simulink model "chua_sim"  (R2022b)
settings: Solver=ode23t  StartTime=0.0  StopTime=Tfin  RelTol=1e-3
values from neighbouring files (symbols this model uses):
  x0 = randn(3,1)*0.2    [main_chua.m]
  xp0 = x0+[0.01;0;0]    [main_chua.m]
undefined symbols (not defined in the file or in its folder): fg_chua
settings Model: Creator=carlonovara  LastModifiedBy=Enf
settings SolverCC: AlgebraicLoopSolver=TrustRegion
settings DataIOCC: ReturnWorkspaceOutputs=off
settings DebuggingCC: UnconnectedInputMsg=warning  UnconnectedOutputMsg=warning  UnconnectedLineMsg=warning  SFMachineParentedDataDiag=warning  ArithmeticOperatorsInVariantConditions=warning
settings ModelReferenceCC: EnableRefExpFcnMdlSchedulingChecks=on
settings SFSimCC: SimUseLocalCustomCode=off  CustomCodeUndefinedFunction=UseInterfaceOnly
settings RTWCC: RTWUseLocalCustomCode=off
settings CodeAppCC: StateflowObjectComments=on

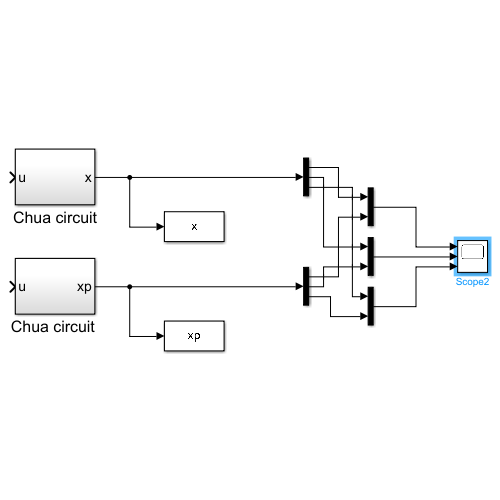
[thumbnail: Simulink's stored preview of the top-level diagram]
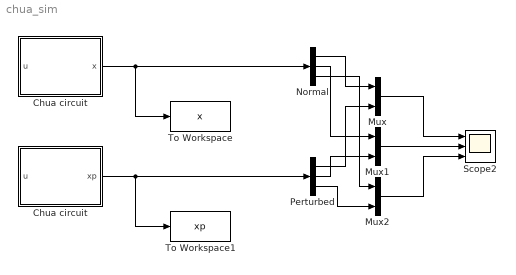
== system chua_sim ==
  Chua circuit : Subsystem
  "Chua circuit " : Subsystem
  Mux : Mux  Inputs=2
  Mux1 : Mux  Inputs=2
  Mux2 : Mux  Inputs=2
  Normal : Demux  Outputs=3
  Perturbed : Demux  Outputs=3
  Scope2 : Scope  NumInputPorts=3
  To Workspace : ToWorkspace  VariableName=x  SampleTime=-1
  To Workspace1 : ToWorkspace  VariableName=xp  SampleTime=-1
  wires:
  Chua circuit/1(x) -> To Workspace/1, Normal/1
  "Chua circuit "/1(xp) -> To Workspace1/1, Perturbed/1
  Mux/1 -> Scope2/1
  Mux1/1 -> Scope2/2
  Mux2/1 -> Scope2/3
  Normal/1 -> Mux/1
  Perturbed/1 -> Mux/2
  Normal/2 -> Mux1/1
  Perturbed/2 -> Mux1/2
  Normal/3 -> Mux2/1
  Perturbed/3 -> Mux2/2

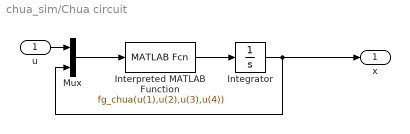
== system chua_sim/Chua circuit ==
  u : Inport
  Integrator : Integrator  InitialCondition=x0
  Interpreted MATLAB Function : MATLABFcn  MATLABFcn=fg_chua(u(1),u(2),u(3),u(4))  OutputDimensions=3
  Mux : Mux  Inputs=2
  x : Outport
  wires:
  u/1 -> Mux/1
  Interpreted MATLAB Function/1 -> Integrator/1
  Integrator/1 -> Mux/2, x/1
  Mux/1 -> Interpreted MATLAB Function/1

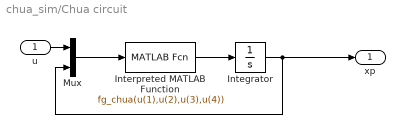
== system chua_sim/Chua circuit  ==
  u : Inport
  Integrator : Integrator  InitialCondition=xp0
  Interpreted MATLAB Function : MATLABFcn  MATLABFcn=fg_chua(u(1),u(2),u(3),u(4))  OutputDimensions=3
  Mux : Mux  Inputs=2
  xp : Outport
  wires:
  Mux/1 -> Interpreted MATLAB Function/1
  Integrator/1 -> Mux/2, xp/1
  Interpreted MATLAB Function/1 -> Integrator/1
  u/1 -> Mux/1
